simulink model "npc_controller"  (R2022a)
settings: Solver=FixedStepDiscrete  StartTime=0.0  StopTime=20  RelTol=1e-3  EnableMultiTasking=on
values from neighbouring files (symbols this model uses):
  Tsw = 1.5E-5    [param.sldd]
undefined symbols (not defined in the file or in its folder): CAN_O_INT, CANA_BASE, Down, GPTRIP1SEL, GPTRIP2SEL, GPTRIP3SEL, TZ1, TZ2, TZ3, Up
libraries: simulink x153, hdlsllib x90, c2802xlib x34, c2837xDlib x18, c280xlib x12, canmsglib x9, c2838xlib x8, idelinklib_common x3, c2806xlib x2, slpidlib x2, c28004xlib x2, c281xlib x2
(part 27 of 45)

== system npc_controller/CONTROL/STATE-MACHINE/CPU_CONTROL_750_A2_precharge_pfc_ok2_OL SS1/updateSequencePhA/pol_final1/pol_vxn ==
  vxn : Inport
  Action Port : ActionPort
  Out1 : Outport
  wires:
  vxn/1 -> Out1/1

== system npc_controller/CONTROL/STATE-MACHINE/CPU_CONTROL_750_A2_precharge_pfc_ok2_OL SS1/updateSequencePhA/pol_final1/prot ==
  note: Note:
      |
      | Function PWM # GPIO # LAUNCHPAD PIN #
      |
      | Synci EPWM1A GPIO0 J4.40
      | EPWM1B GPIO1 J4.39
      |
      | TZ GPIO62 XX
      |
      | a_s1 EPWM6B GPIO11 J8.75
      | a_s2 EPWM7B GPIO13 XX
      | a_s3 EPWM6A GPIO10 J8.76
      | a_s4 EPWM7A GPIO12 XX
      |
      | b_s1 EPWM8B GPIO15 J8.73
      | b_s2 EPWM9B GPIO17 XX
      | b_s3 EPWM8A GPIO14 J8.74
      | b_s4 EPWM9A GPIO16 J4.33
      |
      | c_s1 EPWM10B GPIO19 J1.3
      | c_s2 EPWM11B GPIO21 XX
      | c_s3 EPWM10A GPIO18 J1.4
      | c_s4 EPWM11A GPIO20 XX
  note: /*Force PWM to LOW*/
      | EPwm6Regs.AQCSFRC.bit.CSFA = (uint16_T)(0b01);
      | EPwm6Regs.AQCSFRC.bit.CSFB = (uint16_T)(0b01);
      | EPwm7Regs.AQCSFRC.bit.CSFA = (uint16_T)(0b01);
      | EPwm7Regs.AQCSFRC.bit.CSFB = (uint16_T)(0b01);
      | EPwm8Regs.AQCSFRC.bit.CSFA = (uint16_T)(0b01);
      | EPwm8Regs.AQCSFRC.bit.CSFB = (uint16_T)(0b01);
      | EPwm9Regs.AQCSFRC.bit.CSFA = (uint16_T)(0b01);
      | EPwm9Regs.AQCSFRC.bit.CSFB = (uint16_T)(0b01);
      | EPwm10Regs.AQCSFRC.bit.CSFA = (uint16_T)(0b01);
      | EPwm10Regs.AQCSFRC.bit.CSFB = (uint16_T)(0b01);
      | EPwm11Regs.AQCSFRC.bit.CSFA = (uint16_T)(0b01);
      | EPwm11Regs.AQCSFRC.bit.CSFB = (uint16_T)(0b01);
  note: Note:
      | AQCSFRC
      | 0b00 - disables forced PWM
      | 0b01 - forces PWM to LOW
      | 0b10 - forces PWM to  HIGH
  Action Port : ActionPort
  Constant : Constant  Value=0  OutDataTypeStr=uint8  SampleTime=-1
  System Outputs : Subsystem  mask(System Outputs){ShowInLibBrowser=0}
      mask prompts: ShowInLibBrowser "Simulink:masks:CustCodeMaskParam1_MP"
      settings: CopyFcn=cccopyfcn(gcb)  OpenFcn=ccopenfcn('System Outputs Function')
      mask Help: eval('feval(''rtwprivate'',''rtwhelpview'',''rtw_sys_outputs_block'')');
      mask Display: disp('System\nOutputs');
  Out1 : Outport
  wires:
  Constant/1 -> Out1/1

== system npc_controller/CONTROL/STATE-MACHINE/CPU_CONTROL_750_A2_precharge_pfc_ok2_OL SS1/updateSequencePhA/pol_ix1/neg ==
  Action Port : ActionPort
  Constant : Constant  Value=2  OutDataTypeStr=uint8  SampleTime=-1
  Out1 : Outport
  wires:
  Constant/1 -> Out1/1

== system npc_controller/CONTROL/STATE-MACHINE/CPU_CONTROL_750_A2_precharge_pfc_ok2_OL SS1/updateSequencePhA/pol_ix1/pos ==
  Action Port : ActionPort
  Constant : Constant  OutDataTypeStr=uint8  SampleTime=-1
  Out1 : Outport
  wires:
  Constant/1 -> Out1/1

== system npc_controller/CONTROL/STATE-MACHINE/CPU_CONTROL_750_A2_precharge_pfc_ok2_OL SS1/updateSequencePhA/pol_ix1/zero ==
  Action Port : ActionPort
  Constant : Constant  Value=0  OutDataTypeStr=uint8  SampleTime=-1
  Out1 : Outport
  wires:
  Constant/1 -> Out1/1

== system npc_controller/CONTROL/STATE-MACHINE/CPU_CONTROL_750_A2_precharge_pfc_ok2_OL SS1/updateSequencePhA/pol_vxn1/neg ==
  note: EPwm2Regs.AQCSFRC.bit.CSFA = (uint16_T)(0b01);
      | EPwm7Regs.AQCSFRC.bit.CSFB = (uint16_T)(0b00);
      | EPwm2Regs.AQCSFRC.bit.CSFB = (uint16_T)(0b10);
      | EPwm7Regs.AQCSFRC.bit.CSFA = (uint16_T)(0b01);
  note: Note:
      | AQCSFRC
      | 0b00 - disables forced PWM
      | 0b01 - forces PWM to LOW
      | 0b10 - forces PWM to  HIGH
  note: Note:
      |
      | Function PWM # GPIO # LAUNCHPAD PIN #
      |
      | Synci EPWM1A GPIO0 J4.40
      | EPWM1B GPIO1 J4.39
      |
      | ORPS EPMW2A GPIO2 J4.38
      | EPWM2B GPIO3 J4.37
      |
      | RELAY EPWM3A GPIO4 J4.36
      |
      | TZ GPIO62 XX
      |
      | a_s1 EPWM6A GPIO10 J8.76
      | a_s2 EPWM7B GPIO13 XX
      | a_s3 EPWM6B GPIO11 J8.75
      | a_s4 EPWM7A GPIO12 XX
      |
      | b_s1 EPWM8B GPIO15 J8.73
      | b_s2 EPWM9B GPIO17 XX
      | b_s3 EPWM8A GPIO14 J8.74
      | b_s4 EPWM9A GPIO16 J4.33
      |
      | c_s1 EPWM10B GPIO19 J1.3
      | c_s2 EPWM11B GPIO21 XX
      | c_s3 EPWM10A GPIO18 J1.4
      | c_s4 EPWM11A GPIO20 XX
  Action Port : ActionPort
  Constant : Constant  Value=2  OutDataTypeStr=uint8  SampleTime=-1
  System Outputs1 : Subsystem  mask(System Outputs){ShowInLibBrowser=0}
      mask prompts: ShowInLibBrowser "Simulink:masks:CustCodeMaskParam1_MP"
      settings: CopyFcn=cccopyfcn(gcb)  OpenFcn=ccopenfcn('System Outputs Function')
      mask Help: eval('feval(''rtwprivate'',''rtwhelpview'',''rtw_sys_outputs_block'')');
      mask Display: disp('System\nOutputs');
  Out1 : Outport
  wires:
  Constant/1 -> Out1/1

== system npc_controller/CONTROL/STATE-MACHINE/CPU_CONTROL_750_A2_precharge_pfc_ok2_OL SS1/updateSequencePhA/pol_vxn1/pos ==
  note: Note:
      | AQCSFRC
      | 0b00 - disables forced PWM
      | 0b01 - forces PWM to LOW
      | 0b10 - forces PWM to  HIGH
  note: EPwm2Regs.AQCSFRC.bit.CSFA = (uint16_T)(0b01);
      | EPwm7Regs.AQCSFRC.bit.CSFB = (uint16_T)(0b10);
      | EPwm2Regs.AQCSFRC.bit.CSFB = (uint16_T)(0b00);
      | EPwm7Regs.AQCSFRC.bit.CSFA = (uint16_T)(0b01);
  note: Note:
      |
      | Function PWM # GPIO # LAUNCHPAD PIN #
      |
      | Synci EPWM1A GPIO0 J4.40
      | EPWM1B GPIO1 J4.39
      |
      | ORPS EPMW2A GPIO2 J4.38
      | EPWM2B GPIO3 J4.37
      |
      | RELAY EPWM3A GPIO4 J4.36
      |
      | TZ GPIO62 XX
      |
      | a_s1 EPWM6A GPIO10 J8.76
      | a_s2 EPWM7B GPIO13 XX
      | a_s3 EPWM6B GPIO11 J8.75
      | a_s4 EPWM7A GPIO12 XX
      |
      | b_s1 EPWM8B GPIO15 J8.73
      | b_s2 EPWM9B GPIO17 XX
      | b_s3 EPWM8A GPIO14 J8.74
      | b_s4 EPWM9A GPIO16 J4.33
      |
      | c_s1 EPWM10B GPIO19 J1.3
      | c_s2 EPWM11B GPIO21 XX
      | c_s3 EPWM10A GPIO18 J1.4
      | c_s4 EPWM11A GPIO20 XX
  Action Port : ActionPort
  Constant : Constant  OutDataTypeStr=uint8  SampleTime=-1
  System Outputs1 : Subsystem  mask(System Outputs){ShowInLibBrowser=0}
      mask prompts: ShowInLibBrowser "Simulink:masks:CustCodeMaskParam1_MP"
      settings: CopyFcn=cccopyfcn(gcb)  OpenFcn=ccopenfcn('System Outputs Function')
      mask Help: eval('feval(''rtwprivate'',''rtwhelpview'',''rtw_sys_outputs_block'')');
      mask Display: disp('System\nOutputs');
  Out1 : Outport
  wires:
  Constant/1 -> Out1/1

== system npc_controller/CONTROL/STATE-MACHINE/CPU_CONTROL_750_A2_precharge_pfc_ok2_OL SS1/updateSequencePhA/pol_vxn1/zero ==
  note: /*Force PWM to LOW*/
      | EPwm2Regs.AQCSFRC.bit.CSFA = (uint16_T)(0b01);
      | EPwm7Regs.AQCSFRC.bit.CSFB = (uint16_T)(0b01);
      | EPwm2Regs.AQCSFRC.bit.CSFB = (uint16_T)(0b01);
      | EPwm7Regs.AQCSFRC.bit.CSFA = (uint16_T)(0b01);
  note: Note:
      | AQCSFRC
      | 0b00 - disables forced PWM
      | 0b01 - forces PWM to LOW
      | 0b10 - forces PWM to  HIGH
  note: Note:
      |
      | Function PWM # GPIO # LAUNCHPAD PIN #
      |
      | Synci EPWM1A GPIO0 J4.40
      | EPWM1B GPIO1 J4.39
      |
      | ORPS EPMW2A GPIO2 J4.38
      | EPWM2B GPIO3 J4.37
      |
      | RELAY EPWM3A GPIO4 J4.36
      |
      | TZ GPIO62 XX
      |
      | a_s1 EPWM6A GPIO10 J8.76
      | a_s2 EPWM7B GPIO13 XX
      | a_s3 EPWM6B GPIO11 J8.75
      | a_s4 EPWM7A GPIO12 XX
      |
      | b_s1 EPWM8B GPIO15 J8.73
      | b_s2 EPWM9B GPIO17 XX
      | b_s3 EPWM8A GPIO14 J8.74
      | b_s4 EPWM9A GPIO16 J4.33
      |
      | c_s1 EPWM10B GPIO19 J1.3
      | c_s2 EPWM11B GPIO21 XX
      | c_s3 EPWM10A GPIO18 J1.4
      | c_s4 EPWM11A GPIO20 XX
  Action Port : ActionPort
  Constant : Constant  Value=0  OutDataTypeStr=uint8  SampleTime=-1
  System Outputs1 : Subsystem  mask(System Outputs){ShowInLibBrowser=0}
      mask prompts: ShowInLibBrowser "Simulink:masks:CustCodeMaskParam1_MP"
      settings: CopyFcn=cccopyfcn(gcb)  OpenFcn=ccopenfcn('System Outputs Function')
      mask Help: eval('feval(''rtwprivate'',''rtwhelpview'',''rtw_sys_outputs_block'')');
      mask Display: disp('System\nOutputs');
  Out1 : Outport
  wires:
  Constant/1 -> Out1/1

== system npc_controller/CONTROL/STATE-MACHINE/CPU_CONTROL_750_A2_precharge_pfc_ok2_OL SS1/updateSequencePhB/pol_final1/pol_vxn ==
  vxn : Inport
  Action Port : ActionPort
  Out1 : Outport
  wires:
  vxn/1 -> Out1/1

== system npc_controller/CONTROL/STATE-MACHINE/CPU_CONTROL_750_A2_precharge_pfc_ok2_OL SS1/updateSequencePhB/pol_final1/prot ==
  note: Note:
      |
      | Function PWM # GPIO # LAUNCHPAD PIN #
      |
      | Synci EPWM1A GPIO0 J4.40
      | EPWM1B GPIO1 J4.39
      |
      | TZ GPIO62 XX
      |
      | a_s1 EPWM6B GPIO11 J8.75
      | a_s2 EPWM7B GPIO13 XX
      | a_s3 EPWM6A GPIO10 J8.76
      | a_s4 EPWM7A GPIO12 XX
      |
      | b_s1 EPWM8B GPIO15 J8.73
      | b_s2 EPWM9B GPIO17 XX
      | b_s3 EPWM8A GPIO14 J8.74
      | b_s4 EPWM9A GPIO16 J4.33
      |
      | c_s1 EPWM10B GPIO19 J1.3
      | c_s2 EPWM11B GPIO21 XX
      | c_s3 EPWM10A GPIO18 J1.4
      | c_s4 EPWM11A GPIO20 XX
  note: /*Force PWM to LOW*/
      | EPwm6Regs.AQCSFRC.bit.CSFA = (uint16_T)(0b01);
      | EPwm6Regs.AQCSFRC.bit.CSFB = (uint16_T)(0b01);
      | EPwm7Regs.AQCSFRC.bit.CSFA = (uint16_T)(0b01);
      | EPwm7Regs.AQCSFRC.bit.CSFB = (uint16_T)(0b01);
      | EPwm8Regs.AQCSFRC.bit.CSFA = (uint16_T)(0b01);
      | EPwm8Regs.AQCSFRC.bit.CSFB = (uint16_T)(0b01);
      | EPwm9Regs.AQCSFRC.bit.CSFA = (uint16_T)(0b01);
      | EPwm9Regs.AQCSFRC.bit.CSFB = (uint16_T)(0b01);
      | EPwm10Regs.AQCSFRC.bit.CSFA = (uint16_T)(0b01);
      | EPwm10Regs.AQCSFRC.bit.CSFB = (uint16_T)(0b01);
      | EPwm11Regs.AQCSFRC.bit.CSFA = (uint16_T)(0b01);
      | EPwm11Regs.AQCSFRC.bit.CSFB = (uint16_T)(0b01);
  note: Note:
      | AQCSFRC
      | 0b00 - disables forced PWM
      | 0b01 - forces PWM to LOW
      | 0b10 - forces PWM to  HIGH
  Action Port : ActionPort
  Constant : Constant  Value=0  OutDataTypeStr=uint8  SampleTime=-1
  System Outputs : Subsystem  mask(System Outputs){ShowInLibBrowser=0}
      mask prompts: ShowInLibBrowser "Simulink:masks:CustCodeMaskParam1_MP"
      settings: CopyFcn=cccopyfcn(gcb)  OpenFcn=ccopenfcn('System Outputs Function')
      mask Help: eval('feval(''rtwprivate'',''rtwhelpview'',''rtw_sys_outputs_block'')');
      mask Display: disp('System\nOutputs');
  Out1 : Outport
  wires:
  Constant/1 -> Out1/1

== system npc_controller/CONTROL/STATE-MACHINE/CPU_CONTROL_750_A2_precharge_pfc_ok2_OL SS1/updateSequencePhB/pol_ix1/neg ==
  Action Port : ActionPort
  Constant : Constant  Value=2  OutDataTypeStr=uint8  SampleTime=-1
  Out1 : Outport
  wires:
  Constant/1 -> Out1/1

== system npc_controller/CONTROL/STATE-MACHINE/CPU_CONTROL_750_A2_precharge_pfc_ok2_OL SS1/updateSequencePhB/pol_ix1/pos ==
  Action Port : ActionPort
  Constant : Constant  OutDataTypeStr=uint8  SampleTime=-1
  Out1 : Outport
  wires:
  Constant/1 -> Out1/1

== system npc_controller/CONTROL/STATE-MACHINE/CPU_CONTROL_750_A2_precharge_pfc_ok2_OL SS1/updateSequencePhB/pol_ix1/zero ==
  Action Port : ActionPort
  Constant : Constant  Value=0  OutDataTypeStr=uint8  SampleTime=-1
  Out1 : Outport
  wires:
  Constant/1 -> Out1/1

== system npc_controller/CONTROL/STATE-MACHINE/CPU_CONTROL_750_A2_precharge_pfc_ok2_OL SS1/updateSequencePhB/pol_vxn1/neg ==
  note: Note:
      |
      | Function PWM # GPIO # LAUNCHPAD PIN #
      |
      | Synci EPWM1A GPIO0 J4.40
      | EPWM1B GPIO1 J4.39
      |
      | TZ GPIO62 XX
      |
      | a_s1 EPWM6B GPIO11 J8.75
      | a_s2 EPWM7B GPIO13 XX
      | a_s3 EPWM6A GPIO10 J8.76
      | a_s4 EPWM7A GPIO12 XX
      |
      | b_s1 EPWM8B GPIO15 J8.73
      | b_s2 EPWM9B GPIO17 XX
      | b_s3 EPWM8A GPIO14 J8.74
      | b_s4 EPWM9A GPIO16 J4.33
      |
      | c_s1 EPWM10B GPIO19 J1.3
      | c_s2 EPWM11B GPIO21 XX
      | c_s3 EPWM10A GPIO18 J1.4
      | c_s4 EPWM11A GPIO20 XX
  note: Note:
      | AQCSFRC
      | 0b00 - disables forced PWM
      | 0b01 - forces PWM to LOW
      | 0b10 - forces PWM to  HIGH
  note: EPwm8Regs.AQCSFRC.bit.CSFB = (uint16_T)(0b01);
      | EPwm9Regs.AQCSFRC.bit.CSFB = (uint16_T)(0b00);
      | EPwm8Regs.AQCSFRC.bit.CSFA = (uint16_T)(0b10);
      | EPwm9Regs.AQCSFRC.bit.CSFA = (uint16_T)(0b01);
  Action Port : ActionPort
  Constant : Constant  Value=2  OutDataTypeStr=uint8  SampleTime=-1
  System Outputs1 : Subsystem  mask(System Outputs){ShowInLibBrowser=0}
      mask prompts: ShowInLibBrowser "Simulink:masks:CustCodeMaskParam1_MP"
      settings: CopyFcn=cccopyfcn(gcb)  OpenFcn=ccopenfcn('System Outputs Function')
      mask Help: eval('feval(''rtwprivate'',''rtwhelpview'',''rtw_sys_outputs_block'')');
      mask Display: disp('System\nOutputs');
  Out1 : Outport
  wires:
  Constant/1 -> Out1/1

== system npc_controller/CONTROL/STATE-MACHINE/CPU_CONTROL_750_A2_precharge_pfc_ok2_OL SS1/updateSequencePhB/pol_vxn1/pos ==
  note: Note:
      | AQCSFRC
      | 0b00 - disables forced PWM
      | 0b01 - forces PWM to LOW
      | 0b10 - forces PWM to  HIGH
  note: Note:
      |
      | Function PWM # GPIO # LAUNCHPAD PIN #
      |
      | Synci EPWM1A GPIO0 J4.40
      | EPWM1B GPIO1 J4.39
      |
      | TZ GPIO62 XX
      |
      | a_s1 EPWM6B GPIO11 J8.75
      | a_s2 EPWM7B GPIO13 XX
      | a_s3 EPWM6A GPIO10 J8.76
      | a_s4 EPWM7A GPIO12 XX
      |
      | b_s1 EPWM8B GPIO15 J8.73
      | b_s2 EPWM9B GPIO17 XX
      | b_s3 EPWM8A GPIO14 J8.74
      | b_s4 EPWM9A GPIO16 J4.33
      |
      | c_s1 EPWM10B GPIO19 J1.3
      | c_s2 EPWM11B GPIO21 XX
      | c_s3 EPWM10A GPIO18 J1.4
      | c_s4 EPWM11A GPIO20 XX
  note: EPwm8Regs.AQCSFRC.bit.CSFB = (uint16_T)(0b01);
      | EPwm9Regs.AQCSFRC.bit.CSFB = (uint16_T)(0b10);
      | EPwm8Regs.AQCSFRC.bit.CSFA = (uint16_T)(0b00);
      | EPwm9Regs.AQCSFRC.bit.CSFA = (uint16_T)(0b01);
  Action Port : ActionPort
  Constant : Constant  OutDataTypeStr=uint8  SampleTime=-1
  System Outputs1 : Subsystem  mask(System Outputs){ShowInLibBrowser=0}
      mask prompts: ShowInLibBrowser "Simulink:masks:CustCodeMaskParam1_MP"
      settings: CopyFcn=cccopyfcn(gcb)  OpenFcn=ccopenfcn('System Outputs Function')
      mask Help: eval('feval(''rtwprivate'',''rtwhelpview'',''rtw_sys_outputs_block'')');
      mask Display: disp('System\nOutputs');
  Out1 : Outport
  wires:
  Constant/1 -> Out1/1

== system npc_controller/CONTROL/STATE-MACHINE/CPU_CONTROL_750_A2_precharge_pfc_ok2_OL SS1/updateSequencePhB/pol_vxn1/zero ==
  note: Note:
      |
      | Function PWM # GPIO # LAUNCHPAD PIN #
      |
      | Synci EPWM1A GPIO0 J4.40
      | EPWM1B GPIO1 J4.39
      |
      | TZ GPIO62 XX
      |
      | a_s1 EPWM6B GPIO11 J8.75
      | a_s2 EPWM7B GPIO13 XX
      | a_s3 EPWM6A GPIO10 J8.76
      | a_s4 EPWM7A GPIO12 XX
      |
      | b_s1 EPWM8B GPIO15 J8.73
      | b_s2 EPWM9B GPIO17 XX
      | b_s3 EPWM8A GPIO14 J8.74
      | b_s4 EPWM9A GPIO16 J4.33
      |
      | c_s1 EPWM10B GPIO19 J1.3
      | c_s2 EPWM11B GPIO21 XX
      | c_s3 EPWM10A GPIO18 J1.4
      | c_s4 EPWM11A GPIO20 XX
  note: /*Force PWM to LOW*/
      | EPwm8Regs.AQCSFRC.bit.CSFB = (uint16_T)(0b01);
      | EPwm9Regs.AQCSFRC.bit.CSFB = (uint16_T)(0b01);
      | EPwm8Regs.AQCSFRC.bit.CSFA = (uint16_T)(0b01);
      | EPwm9Regs.AQCSFRC.bit.CSFA = (uint16_T)(0b01);
  note: Note:
      | AQCSFRC
      | 0b00 - disables forced PWM
      | 0b01 - forces PWM to LOW
      | 0b10 - forces PWM to  HIGH
  Action Port : ActionPort
  Constant : Constant  Value=0  OutDataTypeStr=uint8  SampleTime=-1
  System Outputs1 : Subsystem  mask(System Outputs){ShowInLibBrowser=0}
      mask prompts: ShowInLibBrowser "Simulink:masks:CustCodeMaskParam1_MP"
      settings: CopyFcn=cccopyfcn(gcb)  OpenFcn=ccopenfcn('System Outputs Function')
      mask Help: eval('feval(''rtwprivate'',''rtwhelpview'',''rtw_sys_outputs_block'')');
      mask Display: disp('System\nOutputs');
  Out1 : Outport
  wires:
  Constant/1 -> Out1/1

== system npc_controller/CONTROL/STATE-MACHINE/CPU_CONTROL_750_A2_precharge_pfc_ok2_OL SS1/updateSequencePhC/pol_final1/pol_vxn ==
  vxn : Inport
  Action Port : ActionPort
  Out1 : Outport
  wires:
  vxn/1 -> Out1/1

== system npc_controller/CONTROL/STATE-MACHINE/CPU_CONTROL_750_A2_precharge_pfc_ok2_OL SS1/updateSequencePhC/pol_final1/prot ==
  note: Note:
      |
      | Function PWM # GPIO # LAUNCHPAD PIN #
      |
      | Synci EPWM1A GPIO0 J4.40
      | EPWM1B GPIO1 J4.39
      |
      | TZ GPIO62 XX
      |
      | a_s1 EPWM6B GPIO11 J8.75
      | a_s2 EPWM7B GPIO13 XX
      | a_s3 EPWM6A GPIO10 J8.76
      | a_s4 EPWM7A GPIO12 XX
      |
      | b_s1 EPWM8B GPIO15 J8.73
      | b_s2 EPWM9B GPIO17 XX
      | b_s3 EPWM8A GPIO14 J8.74
      | b_s4 EPWM9A GPIO16 J4.33
      |
      | c_s1 EPWM10B GPIO19 J1.3
      | c_s2 EPWM11B GPIO21 XX
      | c_s3 EPWM10A GPIO18 J1.4
      | c_s4 EPWM11A GPIO20 XX
  note: /*Force PWM to LOW*/
      | EPwm6Regs.AQCSFRC.bit.CSFA = (uint16_T)(0b01);
      | EPwm6Regs.AQCSFRC.bit.CSFB = (uint16_T)(0b01);
      | EPwm7Regs.AQCSFRC.bit.CSFA = (uint16_T)(0b01);
      | EPwm7Regs.AQCSFRC.bit.CSFB = (uint16_T)(0b01);
      | EPwm8Regs.AQCSFRC.bit.CSFA = (uint16_T)(0b01);
      | EPwm8Regs.AQCSFRC.bit.CSFB = (uint16_T)(0b01);
      | EPwm9Regs.AQCSFRC.bit.CSFA = (uint16_T)(0b01);
      | EPwm9Regs.AQCSFRC.bit.CSFB = (uint16_T)(0b01);
      | EPwm10Regs.AQCSFRC.bit.CSFA = (uint16_T)(0b01);
      | EPwm10Regs.AQCSFRC.bit.CSFB = (uint16_T)(0b01);
      | EPwm11Regs.AQCSFRC.bit.CSFA = (uint16_T)(0b01);
      | EPwm11Regs.AQCSFRC.bit.CSFB = (uint16_T)(0b01);
  note: Note:
      | AQCSFRC
      | 0b00 - disables forced PWM
      | 0b01 - forces PWM to LOW
      | 0b10 - forces PWM to  HIGH
  Action Port : ActionPort
  Constant : Constant  Value=0  OutDataTypeStr=uint8  SampleTime=-1
  System Outputs : Subsystem  mask(System Outputs){ShowInLibBrowser=0}
      mask prompts: ShowInLibBrowser "Simulink:masks:CustCodeMaskParam1_MP"
      settings: CopyFcn=cccopyfcn(gcb)  OpenFcn=ccopenfcn('System Outputs Function')
      mask Help: eval('feval(''rtwprivate'',''rtwhelpview'',''rtw_sys_outputs_block'')');
      mask Display: disp('System\nOutputs');
  Out1 : Outport
  wires:
  Constant/1 -> Out1/1

== system npc_controller/CONTROL/STATE-MACHINE/CPU_CONTROL_750_A2_precharge_pfc_ok2_OL SS1/updateSequencePhC/pol_ix1/neg ==
  Action Port : ActionPort
  Constant : Constant  Value=2  OutDataTypeStr=uint8  SampleTime=-1
  Out1 : Outport
  wires:
  Constant/1 -> Out1/1

== system npc_controller/CONTROL/STATE-MACHINE/CPU_CONTROL_750_A2_precharge_pfc_ok2_OL SS1/updateSequencePhC/pol_ix1/pos ==
  Action Port : ActionPort
  Constant : Constant  OutDataTypeStr=uint8  SampleTime=-1
  Out1 : Outport
  wires:
  Constant/1 -> Out1/1

== system npc_controller/CONTROL/STATE-MACHINE/CPU_CONTROL_750_A2_precharge_pfc_ok2_OL SS1/updateSequencePhC/pol_ix1/zero ==
  Action Port : ActionPort
  Constant : Constant  Value=0  OutDataTypeStr=uint8  SampleTime=-1
  Out1 : Outport
  wires:
  Constant/1 -> Out1/1

== system npc_controller/CONTROL/STATE-MACHINE/CPU_CONTROL_750_A2_precharge_pfc_ok2_OL SS1/updateSequencePhC/pol_vxn1/neg ==
  note: Note:
      | AQCSFRC
      | 0b00 - disables forced PWM
      | 0b01 - forces PWM to LOW
      | 0b10 - forces PWM to  HIGH
  note: EPwm10Regs.AQCSFRC.bit.CSFB = (uint16_T)(0b01);
      | EPwm11Regs.AQCSFRC.bit.CSFB = (uint16_T)(0b00);
      | EPwm10Regs.AQCSFRC.bit.CSFA = (uint16_T)(0b10);
      | EPwm11Regs.AQCSFRC.bit.CSFA = (uint16_T)(0b01);
  note: Note:
      |
      | Function PWM # GPIO # LAUNCHPAD PIN #
      |
      | Synci EPWM1A GPIO0 J4.40
      | EPWM1B GPIO1 J4.39
      |
      | TZ GPIO62 XX
      |
      | a_s1 EPWM6B GPIO11 J8.75
      | a_s2 EPWM7B GPIO13 XX
      | a_s3 EPWM6A GPIO10 J8.76
      | a_s4 EPWM7A GPIO12 XX
      |
      | b_s1 EPWM8B GPIO15 J8.73
      | b_s2 EPWM9B GPIO17 XX
      | b_s3 EPWM8A GPIO14 J8.74
      | b_s4 EPWM9A GPIO16 J4.33
      |
      | c_s1 EPWM10B GPIO19 J1.3
      | c_s2 EPWM11B GPIO21 XX
      | c_s3 EPWM10A GPIO18 J1.4
      | c_s4 EPWM11A GPIO20 XX
  Action Port : ActionPort
  Constant : Constant  Value=2  OutDataTypeStr=uint8  SampleTime=-1
  System Outputs1 : Subsystem  mask(System Outputs){ShowInLibBrowser=0}
      mask prompts: ShowInLibBrowser "Simulink:masks:CustCodeMaskParam1_MP"
      settings: CopyFcn=cccopyfcn(gcb)  OpenFcn=ccopenfcn('System Outputs Function')
      mask Help: eval('feval(''rtwprivate'',''rtwhelpview'',''rtw_sys_outputs_block'')');
      mask Display: disp('System\nOutputs');
  Out1 : Outport
  wires:
  Constant/1 -> Out1/1

== system npc_controller/CONTROL/STATE-MACHINE/CPU_CONTROL_750_A2_precharge_pfc_ok2_OL SS1/updateSequencePhC/pol_vxn1/pos ==
  note: EPwm10Regs.AQCSFRC.bit.CSFB = (uint16_T)(0b01);
      | EPwm11Regs.AQCSFRC.bit.CSFB = (uint16_T)(0b10);
      | EPwm10Regs.AQCSFRC.bit.CSFA = (uint16_T)(0b00);
      | EPwm11Regs.AQCSFRC.bit.CSFA = (uint16_T)(0b01);
  note: Note:
      |
      | Function PWM # GPIO # LAUNCHPAD PIN #
      |
      | Synci EPWM1A GPIO0 J4.40
      | EPWM1B GPIO1 J4.39
      |
      | TZ GPIO62 XX
      |
      | a_s1 EPWM6B GPIO11 J8.75
      | a_s2 EPWM7B GPIO13 XX
      | a_s3 EPWM6A GPIO10 J8.76
      | a_s4 EPWM7A GPIO12 XX
      |
      | b_s1 EPWM8B GPIO15 J8.73
      | b_s2 EPWM9B GPIO17 XX
      | b_s3 EPWM8A GPIO14 J8.74
      | b_s4 EPWM9A GPIO16 J4.33
      |
      | c_s1 EPWM10B GPIO19 J1.3
      | c_s2 EPWM11B GPIO21 XX
      | c_s3 EPWM10A GPIO18 J1.4
      | c_s4 EPWM11A GPIO20 XX
  note: Note:
      | AQCSFRC
      | 0b00 - disables forced PWM
      | 0b01 - forces PWM to LOW
      | 0b10 - forces PWM to  HIGH
  Action Port : ActionPort
  Constant : Constant  OutDataTypeStr=uint8  SampleTime=-1
  System Outputs1 : Subsystem  mask(System Outputs){ShowInLibBrowser=0}
      mask prompts: ShowInLibBrowser "Simulink:masks:CustCodeMaskParam1_MP"
      settings: CopyFcn=cccopyfcn(gcb)  OpenFcn=ccopenfcn('System Outputs Function')
      mask Help: eval('feval(''rtwprivate'',''rtwhelpview'',''rtw_sys_outputs_block'')');
      mask Display: disp('System\nOutputs');
  Out1 : Outport
  wires:
  Constant/1 -> Out1/1

== system npc_controller/CONTROL/STATE-MACHINE/CPU_CONTROL_750_A2_precharge_pfc_ok2_OL SS1/updateSequencePhC/pol_vxn1/zero ==
  note: Note:
      | AQCSFRC
      | 0b00 - disables forced PWM
      | 0b01 - forces PWM to LOW
      | 0b10 - forces PWM to  HIGH
  note: /*Force PWM to LOW*/
      | EPwm10Regs.AQCSFRC.bit.CSFB = (uint16_T)(0b01);
      | EPwm11Regs.AQCSFRC.bit.CSFB = (uint16_T)(0b01);
      | EPwm10Regs.AQCSFRC.bit.CSFA = (uint16_T)(0b01);
      | EPwm11Regs.AQCSFRC.bit.CSFA = (uint16_T)(0b01);
  note: Note:
      |
      | Function PWM # GPIO # LAUNCHPAD PIN #
      |
      | Synci EPWM1A GPIO0 J4.40
      | EPWM1B GPIO1 J4.39
      |
      | TZ GPIO62 XX
      |
      | a_s1 EPWM6B GPIO11 J8.75
      | a_s2 EPWM7B GPIO13 XX
      | a_s3 EPWM6A GPIO10 J8.76
      | a_s4 EPWM7A GPIO12 XX
      |
      | b_s1 EPWM8B GPIO15 J8.73
      | b_s2 EPWM9B GPIO17 XX
      | b_s3 EPWM8A GPIO14 J8.74
      | b_s4 EPWM9A GPIO16 J4.33
      |
      | c_s1 EPWM10B GPIO19 J1.3
      | c_s2 EPWM11B GPIO21 XX
      | c_s3 EPWM10A GPIO18 J1.4
      | c_s4 EPWM11A GPIO20 XX
  Action Port : ActionPort
  Constant : Constant  Value=0  OutDataTypeStr=uint8  SampleTime=-1
  System Outputs1 : Subsystem  mask(System Outputs){ShowInLibBrowser=0}
      mask prompts: ShowInLibBrowser "Simulink:masks:CustCodeMaskParam1_MP"
      settings: CopyFcn=cccopyfcn(gcb)  OpenFcn=ccopenfcn('System Outputs Function')
      mask Help: eval('feval(''rtwprivate'',''rtwhelpview'',''rtw_sys_outputs_block'')');
      mask Display: disp('System\nOutputs');
  Out1 : Outport
  wires:
  Constant/1 -> Out1/1

== system npc_controller/CONTROL/STATE-MACHINE/CPU_CONTROL_750_A2_precharge_pfc_ok2_OL SS2/configGrid/FORCE_TZ/1P ==
  note: 1 - Leg A
      | 2 - Leg B
      | 3 - Leg C
      | 4 - All legs
  sinlgeph_config : Inport
  Action Port : ActionPort
  ALL_LEGS : Subsystem  Commented=on  TreatAsAtomicUnit=on
  If : If  IfExpression=u1 == 1  ElseIfExpressions=u1 == 2, u1 == 3, u1 == 4
  LEG_A : Subsystem  TreatAsAtomicUnit=on
  LEG_B : Subsystem  TreatAsAtomicUnit=on
  LEG_C : Subsystem  TreatAsAtomicUnit=on
  wires:
  If/4 -> ALL_LEGS/Action
  If/3 -> LEG_C/Action
  If/2 -> LEG_B/Action
  sinlgeph_config/1 -> If/1
  If/1 -> LEG_A/Action

== system npc_controller/CONTROL/STATE-MACHINE/CPU_CONTROL_750_A2_precharge_pfc_ok2_OL SS2/configGrid/FORCE_TZ/3P3W ==
  note: Note:
      | TZCCTL
      | 0b00 - High impedance
      | 0b01 - Force to HIGH
      | 0b10 - Force to LOW
      | 0b11 - Do nothing
      |
      | AQCSFRC
      | 0b00 - disables forced PWM
      | 0b01 - forces PWM to LOW
      | 0b10 - forces PWM to  HIGH
      |
      | TZFRC.bit.OST
      | 0b0 - Do nothing
      | 0b1 - Force TZ
  note: EALLOW;
      |
      | /*Force TZ*/
      | EPwm6Regs. TZFRC.bit.OST = 0b0; //do nothing
      | EPwm7Regs. TZFRC.bit.OST = 0b0;
      | EPwm8Regs. TZFRC.bit.OST = 0b0;
      | EPwm9Regs. TZFRC.bit.OST = 0b0;
      | EPwm10Regs. TZFRC.bit.OST = 0b0;
      | EPwm11Regs. TZFRC.bit.OST = 0b0;
      |
      | EDIS;
  Action Port : ActionPort
  System Outputs2 : Subsystem  mask(System Outputs){ShowInLibBrowser=0}
      mask prompts: ShowInLibBrowser "Simulink:masks:CustCodeMaskParam1_MP"
      settings: CopyFcn=cccopyfcn(gcb)  OpenFcn=ccopenfcn('System Outputs Function')
      mask Help: eval('feval(''rtwprivate'',''rtwhelpview'',''rtw_sys_outputs_block'')');
      mask Display: disp('System\nOutputs');

== system npc_controller/CONTROL/STATE-MACHINE/CPU_CONTROL_750_A2_precharge_pfc_ok2_OL SS2/configGrid/RESET_TZ/System Outputs2 ==

== system npc_controller/CONTROL/STATE-MACHINE/CPU_CONTROL_750_A2_precharge_pfc_ok2_OL SS2/updateCalib/cnt/IIR Filter2 ==
  note: prev 0.98
  x[n] : Inport
  1 - Lambda : Gain  Gain=1 - 0.95  ParamDataTypeStr=single  OutDataTypeStr=single
  Delay : Delay  DelayLength=1
  Lambda : Gain  Gain=0.95  ParamDataTypeStr=single  OutDataTypeStr=single
  Sum : Sum  Inputs=|++  AccumDataTypeStr=single  OutDataTypeStr=single
  y[n] : Outport
  wires:
  x[n]/1 -> 1 - Lambda/1
  1 - Lambda/1 -> Sum/1
  Sum/1 -> Delay/1, y[n]/1
  Lambda/1 -> Sum/2
  Delay/1 -> Lambda/1

== system npc_controller/CONTROL/STATE-MACHINE/CPU_CONTROL_750_A2_precharge_pfc_ok2_OL SS2/updateCalib/cnt/Subsystem1 ==
  sample : Inport
  Add4 : Sum  AccumDataTypeStr=single  OutDataTypeStr=single
  Cast To Single : DataTypeConversion  OutDataTypeStr=single  SaturateOnIntegerOverflow=off  RndMeth=Floor
  Constant4 : Constant  OutDataTypeStr=single
  Data Store Read4 : DataStoreRead  DataStoreName=cnt_calib  IndexOptions=Index vector (dialog)  Indices=1  OutputSizes=1
  Delay2 : Delay  DelayLength=1
  Divide3 : Product  Inputs=*/  OutDataTypeStr=single
  Divide4 : Product  Inputs=**/  OutDataTypeStr=single
  Subtract1 : Sum  Inputs=+-  AccumDataTypeStr=single  OutDataTypeStr=single
  average : Outport
  wires:
  Constant4/1 -> Subtract1/2
  Divide4/1 -> Add4/1
  Cast To Single/1 -> Subtract1/1, Divide4/3, Divide3/2
  Divide3/1 -> Add4/2
  Subtract1/1 -> Divide4/2
  Delay2/1 -> Divide4/1
  sample/1 -> Divide3/1
  Add4/1 -> average/1, Delay2/1
  Data Store Read4/1 -> Cast To Single/1

== system npc_controller/CONTROL/STATE-MACHINE/CPU_CONTROL_750_A2_precharge_pfc_ok2_OL SS2/updateCalib/cnt/Subsystem2 ==
  sample : Inport
  Add4 : Sum  AccumDataTypeStr=single  OutDataTypeStr=single
  Cast To Single : DataTypeConversion  OutDataTypeStr=single  SaturateOnIntegerOverflow=off  RndMeth=Floor
  Constant4 : Constant  OutDataTypeStr=single
  Data Store Read4 : DataStoreRead  DataStoreName=cnt_calib  IndexOptions=Index vector (dialog)  Indices=1  OutputSizes=1
  Delay2 : Delay  DelayLength=1
  Divide3 : Product  Inputs=*/  OutDataTypeStr=single
  Divide4 : Product  Inputs=**/  OutDataTypeStr=single
  Subtract1 : Sum  Inputs=+-  AccumDataTypeStr=single  OutDataTypeStr=single
  average : Outport
  wires:
  Data Store Read4/1 -> Cast To Single/1
  Add4/1 -> Delay2/1, average/1
  sample/1 -> Divide3/1
  Delay2/1 -> Divide4/1
  Subtract1/1 -> Divide4/2
  Divide3/1 -> Add4/2
  Cast To Single/1 -> Divide3/2, Divide4/3, Subtract1/1
  Divide4/1 -> Add4/1
  Constant4/1 -> Subtract1/2

== system npc_controller/CONTROL/STATE-MACHINE/CPU_CONTROL_750_A2_precharge_pfc_ok2_OL SS2/updateCalib/cnt/Subsystem3 ==
  sample : Inport
  Add4 : Sum  AccumDataTypeStr=single  OutDataTypeStr=single
  Cast To Single : DataTypeConversion  OutDataTypeStr=single  SaturateOnIntegerOverflow=off  RndMeth=Floor
  Constant4 : Constant  OutDataTypeStr=single
  Data Store Read4 : DataStoreRead  DataStoreName=cnt_calib  IndexOptions=Index vector (dialog)  Indices=1  OutputSizes=1
  Delay2 : Delay  DelayLength=1
  Divide3 : Product  Inputs=*/  OutDataTypeStr=single
  Divide4 : Product  Inputs=**/  OutDataTypeStr=single
  Subtract1 : Sum  Inputs=+-  AccumDataTypeStr=single  OutDataTypeStr=single
  average : Outport
  wires:
  Data Store Read4/1 -> Cast To Single/1
  Add4/1 -> Delay2/1, average/1
  sample/1 -> Divide3/1
  Delay2/1 -> Divide4/1
  Subtract1/1 -> Divide4/2
  Divide3/1 -> Add4/2
  Cast To Single/1 -> Divide3/2, Divide4/3, Subtract1/1
  Divide4/1 -> Add4/1
  Constant4/1 -> Subtract1/2

== system npc_controller/CONTROL/STATE-MACHINE/CPU_CONTROL_750_A2_precharge_pfc_ok2_OL SS2/updateCalib/cnt/Subsystem4 ==
  sample : Inport
  Add4 : Sum  AccumDataTypeStr=single  OutDataTypeStr=single
  Cast To Single : DataTypeConversion  OutDataTypeStr=single  SaturateOnIntegerOverflow=off  RndMeth=Floor
  Constant4 : Constant  OutDataTypeStr=single
  Data Store Read4 : DataStoreRead  DataStoreName=cnt_calib  IndexOptions=Index vector (dialog)  Indices=1  OutputSizes=1
  Delay2 : Delay  DelayLength=1
  Divide3 : Product  Inputs=*/  OutDataTypeStr=single
  Divide4 : Product  Inputs=**/  OutDataTypeStr=single
  Subtract1 : Sum  Inputs=+-  AccumDataTypeStr=single  OutDataTypeStr=single
  average : Outport
  wires:
  Constant4/1 -> Subtract1/2
  Divide4/1 -> Add4/1
  Cast To Single/1 -> Subtract1/1, Divide4/3, Divide3/2
  Divide3/1 -> Add4/2
  Subtract1/1 -> Divide4/2
  Delay2/1 -> Divide4/1
  sample/1 -> Divide3/1
  Add4/1 -> average/1, Delay2/1
  Data Store Read4/1 -> Cast To Single/1

== system npc_controller/CONTROL/STATE-MACHINE/CPU_CONTROL_750_A2_precharge_pfc_ok2_OL SS2/updateCalib/cnt/Subsystem5 ==
  sample : Inport
  Add4 : Sum  AccumDataTypeStr=single  OutDataTypeStr=single
  Cast To Single : DataTypeConversion  OutDataTypeStr=single  SaturateOnIntegerOverflow=off  RndMeth=Floor
  Constant4 : Constant  OutDataTypeStr=single
  Data Store Read4 : DataStoreRead  DataStoreName=cnt_calib  IndexOptions=Index vector (dialog)  Indices=1  OutputSizes=1
  Delay2 : Delay  DelayLength=1
  Divide3 : Product  Inputs=*/  OutDataTypeStr=single
  Divide4 : Product  Inputs=**/  OutDataTypeStr=single
  Subtract1 : Sum  Inputs=+-  AccumDataTypeStr=single  OutDataTypeStr=single
  average : Outport
  wires:
  Constant4/1 -> Subtract1/2
  Divide4/1 -> Add4/1
  Cast To Single/1 -> Subtract1/1, Divide4/3, Divide3/2
  Divide3/1 -> Add4/2
  Subtract1/1 -> Divide4/2
  Delay2/1 -> Divide4/1
  sample/1 -> Divide3/1
  Add4/1 -> average/1, Delay2/1
  Data Store Read4/1 -> Cast To Single/1

== system npc_controller/CONTROL/STATE-MACHINE/CPU_CONTROL_750_A2_precharge_pfc_ok2_OL SS2/updateCalib/cnt/Subsystem6 ==
  sample : Inport
  Add4 : Sum  AccumDataTypeStr=single  OutDataTypeStr=single
  Cast To Single : DataTypeConversion  OutDataTypeStr=single  SaturateOnIntegerOverflow=off  RndMeth=Floor
  Constant4 : Constant  OutDataTypeStr=single
  Data Store Read4 : DataStoreRead  DataStoreName=cnt_calib  IndexOptions=Index vector (dialog)  Indices=1  OutputSizes=1
  Delay2 : Delay  DelayLength=1
  Divide3 : Product  Inputs=*/  OutDataTypeStr=single
  Divide4 : Product  Inputs=**/  OutDataTypeStr=single
  Subtract1 : Sum  Inputs=+-  AccumDataTypeStr=single  OutDataTypeStr=single
  average : Outport
  wires:
  Data Store Read4/1 -> Cast To Single/1
  Add4/1 -> Delay2/1, average/1
  sample/1 -> Divide3/1
  Delay2/1 -> Divide4/1
  Subtract1/1 -> Divide4/2
  Divide3/1 -> Add4/2
  Cast To Single/1 -> Divide3/2, Divide4/3, Subtract1/1
  Divide4/1 -> Add4/1
  Constant4/1 -> Subtract1/2

== system npc_controller/CONTROL/STATE-MACHINE/CPU_CONTROL_750_A2_precharge_pfc_ok2_OL SS2/updateCalib/done/AUTO-CALIB_DONE ==
  Trigger : TriggerPort  TriggerType=function-call  VariantControl=(inherit)  PortDimensions=1
  Constant1 : Constant  OutDataTypeStr=boolean  SampleTime=-1
  Constant2 : Constant  OutDataTypeStr=uint16  SampleTime=-1
  Data Store Read : DataStoreRead  DataStoreName=adc_offset_ib_tmp  IndexOptions=Index vector (dialog)  Indices=1  OutputSizes=1
  Data Store Read1 : DataStoreRead  DataStoreName=adc_offset_ic_tmp  IndexOptions=Index vector (dialog)  Indices=1  OutputSizes=1
  Data Store Read2 : DataStoreRead  DataStoreName=adc_offset_va_tmp  IndexOptions=Index vector (dialog)  Indices=1  OutputSizes=1
  Data Store Read3 : DataStoreRead  DataStoreName=adc_offset_vb_tmp  IndexOptions=Index vector (dialog)  Indices=1  OutputSizes=1
  Data Store Read4 : DataStoreRead  DataStoreName=adc_offset_vc_tmp  IndexOptions=Index vector (dialog)  Indices=1  OutputSizes=1
  Data Store Read5 : DataStoreRead  DataStoreName=adc_offset_ia_tmp  IndexOptions=Index vector (dialog)  Indices=1  OutputSizes=1
  Data Store Write : DataStoreWrite  DataStoreName=adc_offset_ib  IndexOptions=Index vector (dialog)  Indices=1  OutputSizes=1
  Data Store Write1 : DataStoreWrite  DataStoreName=adc_offset_ic  IndexOptions=Index vector (dialog)  Indices=1  OutputSizes=1
  Data Store Write2 : DataStoreWrite  DataStoreName=cnt_calib  IndexOptions=Index vector (dialog)  Indices=1  OutputSizes=1
  Data Store Write3 : DataStoreWrite  DataStoreName=adc_offset_va  IndexOptions=Index vector (dialog)  Indices=1  OutputSizes=1
  Data Store Write4 : DataStoreWrite  DataStoreName=adc_offset_vb  IndexOptions=Index vector (dialog)  Indices=1  OutputSizes=1
  Data Store Write5 : DataStoreWrite  DataStoreName=adc_offset_vc  IndexOptions=Index vector (dialog)  Indices=1  OutputSizes=1
  Data Store Write6 : DataStoreWrite  DataStoreName=adc_offset_ia  IndexOptions=Index vector (dialog)  Indices=1  OutputSizes=1
  Scope : Scope
  Out1 : Outport
  wires:
  Data Store Read1/1 -> Data Store Write1/1
  Data Store Read3/1 -> Data Store Write4/1
  Data Store Read4/1 -> Data Store Write5/1
  Data Store Read2/1 -> Data Store Write3/1, Scope/1
  Data Store Read/1 -> Data Store Write/1
  Constant2/1 -> Data Store Write2/1
  Data Store Read5/1 -> Data Store Write6/1
  Constant1/1 -> Out1/1

== system npc_controller/CONTROL/STATE-MACHINE/CPU_CONTROL_750_A2_precharge_pfc_ok2_OL SS2/updateCalib/done/CLEAR_FAULTS ==
  Trigger : TriggerPort  TriggerType=function-call  VariantControl=(inherit)  PortDimensions=1
  Constant1 : Constant  Value=0  OutDataTypeStr=uint16  SampleTime=-1
  Constant3 : Constant  Value=0  OutDataTypeStr=boolean  SampleTime=-1
  Constant4 : Constant  Value=0  OutDataTypeStr=boolean  SampleTime=-1
  Constant5 : Constant  Value=0  OutDataTypeStr=boolean  SampleTime=-1
  Constant6 : Constant  Value=0  OutDataTypeStr=uint16  SampleTime=-1
  Constant7 : Constant  Value=0  OutDataTypeStr=uint16  SampleTime=-1
  Data Store Write1 : DataStoreWrite  DataStoreName=tz_cmpssocp  IndexOptions=Index vector (dialog)  Indices=1  OutputSizes=1
  Data Store Write10 : DataStoreWrite  DataStoreName=tz_ocp  IndexOptions=Index vector (dialog)  Indices=1  OutputSizes=1
  Data Store Write11 : DataStoreWrite  DataStoreName=tz_ovp  IndexOptions=Index vector (dialog)  Indices=1  OutputSizes=1
  Data Store Write7 : DataStoreWrite  DataStoreName=tfv_iphasea  IndexOptions=Index vector (dialog)  Indices=1  OutputSizes=1
  Data Store Write8 : DataStoreWrite  DataStoreName=tfv_iphaseb  IndexOptions=Index vector (dialog)  Indices=1  OutputSizes=1
  Data Store Write9 : DataStoreWrite  DataStoreName=tfv_iphasec  IndexOptions=Index vector (dialog)  Indices=1  OutputSizes=1
  wires:
  Constant7/1 -> Data Store Write11/1
  Constant4/1 -> Data Store Write8/1
  Constant3/1 -> Data Store Write7/1
  Constant5/1 -> Data Store Write9/1
  Constant6/1 -> Data Store Write10/1
  Constant1/1 -> Data Store Write1/1

== system npc_controller/CONTROL/STATE-MACHINE/CPU_CONTROL_750_A2_precharge_pfc_ok2_OL SS2/updateCalib/done/RESET_TZ ==
  note: //npc_controller_DWork.tz_ocp = 0b0;
      |
      | EALLOW;
      |
      | /*Disabled tripzone action*/
      | EPwm2Regs.TZCTL.bit.TZA = (uint16_T)(0b11); //do nothing
      | EPwm2Regs.TZCTL.bit.TZB = (uint16_T)(0b11);
      | EPwm7Regs.TZCTL.bit.TZA = (uint16_T)(0b11);
      | EPwm7Regs.TZCTL.bit.TZB = (uint16_T)(0b11);
      | EPwm8Regs.TZCTL.bit.TZA = (uint16_T)(0b11);
      | EPwm8Regs.TZCTL.bit.TZB = (uint16_T)(0b11);
      | EPwm9Regs.TZCTL.bit.TZA = (uint16_T)(0b11);
      | EPwm9Regs.TZCTL.bit.TZB = (uint16_T)(0b11);
      | EPwm10Regs.TZCTL.bit.TZA = (uint16_T)(0b11);
      | EPwm10Regs.TZCTL.bit.TZB = (uint16_T)(0b11);
      | EPwm11Regs.TZCTL.bit.TZA = (uint16_T)(0b11);
      | EPwm11Regs.TZCTL.bit.TZB = (uint16_T)(0b11);
      |
      | /*Clear grouped OST TZ flags*/
      | EPwm2Regs.TZCLR.bit.OST = 0b1; //clear trip
      | EPwm7Regs.TZCLR.bit.OST = 0b1;
      | EPwm8Regs.TZCLR.bit.OST = 0b1;
      | EPwm9Regs.TZCLR.bit.OST = 0b1;
      | EPwm10Regs.TZCLR.bit.OST = 0b1;
      | EPwm11Regs.TZCLR.bit.OST = 0b1;
      |
      | /*Clear individual OST TZ flags*/
      | EPwm2Regs.TZOSTCLR.bit.OST1 = 0b1; //clear trip
      | EPwm2Regs.TZOSTCLR.bit.OST2 = 0b1;
      | EPwm7Regs.TZOSTCLR.bit.OST1 = 0b1;
      | EPwm7Regs.TZOSTCLR.bit.OST2 = 0b1;
      | EPwm8Regs.TZOSTCLR.bit.OST1 = 0b1;
      | EPwm8Regs.TZOSTCLR.bit.OST2 = 0b1;
      | EPwm9Regs.TZOSTCLR.bit.OST1 = 0b1;
      | EPwm9Regs.TZOSTCLR.bit.OST2 = 0b1;
      | EPwm10Regs.TZOSTCLR.bit.OST1 = 0b1;
      | EPwm10Regs.TZOSTCLR.bit.OST2 = 0b1;
      | EPwm11Regs.TZOSTCLR.bit.OST1 = 0b1;
      | EPwm11Regs.TZOSTCLR.bit.OST2 = 0b1;
      |
      | /*Enable tripzone action*/
      | EPwm2Regs.TZCTL.bit.TZA = (uint16_T)(0b10); //force to LOW
      | EPwm2Regs.TZCTL.bit.TZB = (uint16_T)(0b10);
      | EPwm7Regs.TZCTL.bit.TZA = (uint16_T)(0b10);
      | EPwm7Regs.TZCTL.bit.TZB = (uint16_T)(0b10);
      | EPwm8Regs.TZCTL.bit.TZA = (uint16_T)(0b10);
      | EPwm8Regs.TZCTL.bit.TZB = (uint16_T)(0b10);
      | EPwm9Regs.TZCTL.bit.TZA = (uint16_T)(0b10);
      | EPwm9Regs.TZCTL.bit.TZB = (uint16_T)(0b10);
      | EPwm10Regs.TZCTL.bit.TZA = (uint16_T)(0b10);
      | EPwm10Regs.TZCTL.bit.TZB = (uint16_T)(0b10);
      | EPwm11Regs.TZCTL.bit.TZA = (uint16_T)(0b10);
      | EPwm11Regs.TZCTL.bit.TZB = (uint16_T)(0b10);
      |
      | EDIS;
  note: Note:
      | TZCCTL
      | 0b00 - High impedance
      | 0b01 - Force to HIGH
      | 0b10 - Force to LOW
      | 0b11 - Do nothing
      |
      | AQCSFRC
      | 0b00 - disables forced PWM
      | 0b01 - forces PWM to LOW
      | 0b10 - forces PWM to  HIGH
  note: //npc_controller_DWork.tz_ocp = 0b0;
      |
      | EALLOW;
      |
      | /*Disabled tripzone action*/
      | EPwm2Regs.TZCTL.bit.TZA = (uint16_T)(0b11); //do nothing
      | EPwm2Regs.TZCTL.bit.TZB = (uint16_T)(0b11);
      | EPwm7Regs.TZCTL.bit.TZA = (uint16_T)(0b11);
      | EPwm7Regs.TZCTL.bit.TZB = (uint16_T)(0b11);
      | EPwm8Regs.TZCTL.bit.TZA = (uint16_T)(0b11);
      | EPwm8Regs.TZCTL.bit.TZB = (uint16_T)(0b11);
      | EPwm9Regs.TZCTL.bit.TZA = (uint16_T)(0b11);
      | EPwm9Regs.TZCTL.bit.TZB = (uint16_T)(0b11);
      | EPwm10Regs.TZCTL.bit.TZA = (uint16_T)(0b11);
      | EPwm10Regs.TZCTL.bit.TZB = (uint16_T)(0b11);
      | EPwm11Regs.TZCTL.bit.TZA = (uint16_T)(0b11);
      | EPwm11Regs.TZCTL.bit.TZB = (uint16_T)(0b11);
      |
      | /*Disabled Digital Compare Out A and Out B Event1*/
      | //EPwm2Regs.TZCTL.bit.DCAEVT1 = 0b11; //do nothing
      | //EPwm2Regs.TZCTL.bit.DCBEVT1 = 0b11;
      | //EPwm7Regs.TZCTL.bit.DCAEVT1 = 0b11;
      | //EPwm7Regs.TZCTL.bit.DCBEVT1 = 0b11;
      |
      | //EPwm8Regs.TZCTL.bit.DCAEVT1 = 0b11;
      | //EPwm8Regs.TZCTL.bit.DCBEVT1 = 0b11;
      | //EPwm9Regs.TZCTL.bit.DCAEVT1 = 0b11;
      | //EPwm9Regs.TZCTL.bit.DCBEVT1 = 0b11;
      |
      | //EPwm10Regs.TZCTL.bit.DCAEVT1 = 0b11;
      | //EPwm10Regs.TZCTL.bit.DCBEVT1 = 0b11;
      | //EPwm11Regs.TZCTL.bit.DCAEVT1 = 0b11;
      | //EPwm11Regs.TZCTL.bit.DCBEVT1 = 0b11;
      |
      | /*Disabled Digital Compare Out A and Out B Event1 */
      | EPwm2Regs.TZSEL.bit.DCAEVT1 = 0b0; //disable DCAEVT1 for the ePWM module
      | EPwm2Regs.TZSEL.bit.DCBEVT1 = 0b0;
      | EPwm7Regs.TZSEL.bit.DCAEVT1 = 0b0;
      | EPwm7Regs.TZSEL.bit.DCBEVT1 = 0b0;
      |
      | EPwm8Regs.TZSEL.bit.DCAEVT1 = 0b0;
      | EPwm8Regs.TZSEL.bit.DCBEVT1 = 0b0;
      | EPwm9Regs.TZSEL.bit.DCAEVT1 = 0b0;
      | EPwm9Regs.TZSEL.bit.DCBEVT1 = 0b0;
      |
      | EPwm10Regs.TZSEL.bit.DCAEVT1 = 0b0;
      | EPwm10Regs.TZSEL.bit.DCBEVT1 = 0b0;
      | EPwm11Regs.TZSEL.bit.DCAEVT1 = 0b0;
      | EPwm11Regs.TZSEL.bit.DCBEVT1 = 0b0;
      |
      | /*Clear grouped OST TZ flags*/
      | EPwm2Regs.TZCLR.bit.OST = 0b1; //clear trip
      | EPwm7Regs.TZCLR.bit.OST = 0b1;
      | EPwm8Regs.TZCLR.bit.OST = 0b1;
      | EPwm9Regs.TZCLR.bit.OST = 0b1;
      | EPwm10Regs.TZCLR.bit.OST = 0b1;
      | EPwm11Regs.TZCLR.bit.OST = 0b1;
      |
      | /*Clear Digital Compare Out A and B Event1 flags */
      | EPwm2Regs.TZCLR.bit.DCAEVT1 = 0b1; //clear trip
      | EPwm2Regs.TZCLR.bit.DCBEVT1 = 0b1;
      | EPwm7Regs.TZCLR.bit.DCAEVT1 = 0b1;
      | EPwm7Regs.TZCLR.bit.DCBEVT1 = 0b1;
      |
      | EPwm8Regs.TZCLR.bit.DCAEVT1 = 0b1;
      | EPwm8Regs.TZCLR.bit.DCBEVT1 = 0b1;
      | EPwm9Regs.TZCLR.bit.DCAEVT1 = 0b1;
      | EPwm9Regs.TZCLR.bit.DCBEVT1 = 0b1;
      |
      | EPwm10Regs.TZCLR.bit.DCAEVT1 = 0b1;
      | EPwm10Regs.TZCLR.bit.DCBEVT1 = 0b1;
      | EPwm11Regs.TZCLR.bit.DCAEVT1 = 0b1;
      | EPwm11Regs.TZCLR.bit.DCBEVT1 = 0b1;
      |
      | /*Enabled Digital Compare Out A and Out B Event1 */
      | EPwm2Regs.TZSEL.bit.DCAEVT1 = 0b1; //enabled DCAEVT1 for the ePWM module
      | EPwm2Regs.TZSEL.bit.DCBEVT1 = 0b1;
      | EPwm7Regs.TZSEL.bit.DCAEVT1 = 0b1;
      | EPwm7Regs.TZSEL.bit.DCBEVT1 = 0b1;
      |
      | EPwm8Regs.TZSEL.bit.DCAEVT1 = 0b1;
      | EPwm8Regs.TZSEL.bit.DCBEVT1 = 0b1;
      | EPwm9Regs.TZSEL.bit.DCAEVT1 = 0b1;
      | EPwm9Regs.TZSEL.bit.DCBEVT1 = 0b1;
      |
      | EPwm10Regs.TZSEL.bit.DCAEVT1 = 0b1;
      | EPwm10Regs.TZSEL.bit.DCBEVT1 = 0b1;
      | EPwm11Regs.TZSEL.bit.DCAEVT1 = 0b1;
      | EPwm11Regs.TZSEL.bit.DCBEVT1 = 0b1;
      |
      | /*Clear individual OST TZ flags*/
      | EPwm2Regs.TZOSTCLR.bit.OST1 = 0b1; //clear trip
      | EPwm2Regs.TZOSTCLR.bit.OST2 = 0b1;
      | EPwm7Regs.TZOSTCLR.bit.OST1 = 0b1;
      | EPwm7Regs.TZOSTCLR.bit.OST2 = 0b1;
      | EPwm8Regs.TZOSTCLR.bit.OST1 = 0b1;
      | EPwm8Regs.TZOSTCLR.bit.OST2 = 0b1;
      | EPwm9Regs.TZOSTCLR.bit.OST1 = 0b1;
      | EPwm9Regs.TZOSTCLR.bit.OST2 = 0b1;
      | EPwm10Regs.TZOSTCLR.bit.OST1 = 0b1;
      | EPwm10Regs.TZOSTCLR.bit.OST2 = 0b1;
      | EPwm11Regs.TZOSTCLR.bit.OST1 = 0b1;
      | EPwm11Regs.TZOSTCLR.bit.OST2 = 0b1;
      |
      | /*Enable tripzone action*/
      | EPwm2Regs.TZCTL.bit.TZA = (uint16_T)(0b10); //force to LOW
      | EPwm2Regs.TZCTL.bit.TZB = (uint16_T)(0b10);
      | EPwm7Regs.TZCTL.bit.TZA = (uint16_T)(0b10);
      | EPwm7Regs.TZCTL.bit.TZB = (uint16_T)(0b10);
      | EPwm8Regs.TZCTL.bit.TZA = (uint16_T)(0b10);
      | EPwm8Regs.TZCTL.bit.TZB = (uint16_T)(0b10);
      | EPwm9Regs.TZCTL.bit.TZA = (uint16_T)(0b10);
      | EPwm9Regs.TZCTL.bit.TZB = (uint16_T)(0b10);
      | EPwm10Regs.TZCTL.bit.TZA = (uint16_T)(0b10);
      | EPwm10Regs.TZCTL.bit.TZB = (uint16_T)(0b10);
      | EPwm11Regs.TZCTL.bit.TZA = (uint16_T)(0b10);
      | EPwm11Regs.TZCTL.bit.TZB = (uint16_T)(0b10);
      |
      | /*Enabled Digital Compare Out A and Out B Event1*/
      | //EPwm2Regs.TZCTL.bit.DCAEVT1 = 0b10; //force to LOW
      | //EPwm2Regs.TZCTL.bit.DCBEVT1 = 0b10;
      | //EPwm7Regs.TZCTL.bit.DCAEVT1 = 0b10;
      | //EPwm7Regs.TZCTL.bit.DCBEVT1 = 0b10;
      |
      | //EPwm8Regs.TZCTL.bit.DCAEVT1 = 0b10;
      | //EPwm8Regs.TZCTL.bit.DCBEVT1 = 0b10;
      | //EPwm9Regs.TZCTL.bit.DCAEVT1 = 0b10;
      | //EPwm9Regs.TZCTL.bit.DCBEVT1 = 0b10;
      |
      | //EPwm10Regs.TZCTL.bit.DCAEVT1 = 0b10;
      | //EPwm10Regs.TZCTL.bit.DCBEVT1 = 0b10;
      | //EPwm11Regs.TZCTL.bit.DCAEVT1 = 0b10;
      | //EPwm11Regs.TZCTL.bit.DCBEVT1 = 0b10;
      |
      | EDIS;
  Trigger : TriggerPort  TriggerType=function-call  VariantControl=(inherit)  PortDimensions=1
  System Outputs1 : Subsystem  mask(System Outputs){ShowInLibBrowser=0}
      mask prompts: ShowInLibBrowser "Simulink:masks:CustCodeMaskParam1_MP"
      settings: CopyFcn=cccopyfcn(gcb)  OpenFcn=ccopenfcn('System Outputs Function')
      mask Help: eval('feval(''rtwprivate'',''rtwhelpview'',''rtw_sys_outputs_block'')');
      mask Display: disp('System\nOutputs');
  System Outputs2 : Subsystem  Commented=on  mask(System Outputs){ShowInLibBrowser=0}
      mask prompts: ShowInLibBrowser "Simulink:masks:CustCodeMaskParam1_MP"
      settings: CopyFcn=cccopyfcn(gcb)  OpenFcn=ccopenfcn('System Outputs Function')
      mask Help: eval('feval(''rtwprivate'',''rtwhelpview'',''rtw_sys_outputs_block'')');
      mask Display: disp('System\nOutputs');

== system npc_controller/CONTROL/STATE-MACHINE/CPU_CONTROL_750_A2_precharge_pfc_ok2_OL SS2/updatePll3p/PLL/SRF_PLL ==
  Vabc : Inport
  Demux1 : Demux  Outputs=3
  Gain : Gain  Commented=on  Gain=1/(2*pi)
  Integrator : Subsystem
  Memory : Memory  InheritSampleTime=on  LinearizeAsDelay=on
  PI : Subsystem
  Subsystem1 : Subsystem  Commented=on
  Sum1 : Sum  Inputs=|++  AccumDataTypeStr=single  OutDataTypeStr=single
  abc to dq : Subsystem
  f0 : Constant  Value=2*pi*50  OutDataTypeStr=fixdt('single', 'DataTypeOverride', 'Off')
  SinVal : Outport  VectorParamsAs1DForOutWhenUnconnected=off
  CosVal : Outport  Port=2  VectorParamsAs1DForOutWhenUnconnected=off
  theta : Outport  Port=3  OutDataTypeStr=single  VectorParamsAs1DForOutWhenUnconnected=off
  wires:
  Demux1/3 -> abc to dq/3(c)
  Demux1/2 -> abc to dq/2(b)
  Demux1/1 -> abc to dq/1(a)
  Sum1/1 -> Integrator/1(PI Out), Gain/1
  PI/1(PI Out) -> Sum1/1
  Gain/1 -> Subsystem1/1(x[n])  "Freq_Unf"
  f0/1 -> Sum1/2
  abc to dq/1(q) -> PI/1(Vq)
  Integrator/1(wt) -> theta/1, Memory/1
  Memory/1 -> abc to dq/4(wt)
  Vabc/1 -> Demux1/1

== system npc_controller/CONTROL/STATE-MACHINE/CPU_CONTROL_750_A2_precharge_pfc_ok2_OL SS2/updatePll3p/PLL/Subsystem ==
  In1 : Inport
  Cast To Single : DataTypeConversion  OutDataTypeStr=single  SaturateOnIntegerOverflow=off  RndMeth=Floor
  Constant2 : Constant  Value=0
  GreaterThan1 : RelationalOperator  Operator=>  OutDataTypeStr=boolean  RndMeth=Simplest  InputSameDT=off
  Initialize at Zero Crossing : Subsystem  TreatAsAtomicUnit=on
  Out1 : Outport
  wires:
  Cast To Single/1 -> Out1/1
  In1/1 -> GreaterThan1/1
  Initialize at Zero Crossing/1(Out1) -> Cast To Single/1
  Constant2/1 -> GreaterThan1/2
  GreaterThan1/1 -> Initialize at Zero Crossing/1(In1), Initialize at Zero Crossing/Trigger

== system npc_controller/CONTROL/STATE-MACHINE/CPU_CONTROL_750_A2_precharge_pfc_ok2_OL SS2/updateSequencePhA/pol_final1/pol_vxn ==
  vxn : Inport
  Action Port : ActionPort
  Out1 : Outport
  wires:
  vxn/1 -> Out1/1

== system npc_controller/CONTROL/STATE-MACHINE/CPU_CONTROL_750_A2_precharge_pfc_ok2_OL SS2/updateSequencePhA/pol_final1/prot ==
  note: Note:
      | AQCSFRC
      | 0b00 - disables forced PWM
      | 0b01 - forces PWM to LOW
      | 0b10 - forces PWM to  HIGH
  note: /*Force PWM to LOW*/
      | EPwm6Regs.AQCSFRC.bit.CSFA = (uint16_T)(0b01);
      | EPwm6Regs.AQCSFRC.bit.CSFB = (uint16_T)(0b01);
      | EPwm7Regs.AQCSFRC.bit.CSFA = (uint16_T)(0b01);
      | EPwm7Regs.AQCSFRC.bit.CSFB = (uint16_T)(0b01);
      | EPwm8Regs.AQCSFRC.bit.CSFA = (uint16_T)(0b01);
      | EPwm8Regs.AQCSFRC.bit.CSFB = (uint16_T)(0b01);
      | EPwm9Regs.AQCSFRC.bit.CSFA = (uint16_T)(0b01);
      | EPwm9Regs.AQCSFRC.bit.CSFB = (uint16_T)(0b01);
      | EPwm10Regs.AQCSFRC.bit.CSFA = (uint16_T)(0b01);
      | EPwm10Regs.AQCSFRC.bit.CSFB = (uint16_T)(0b01);
      | EPwm11Regs.AQCSFRC.bit.CSFA = (uint16_T)(0b01);
      | EPwm11Regs.AQCSFRC.bit.CSFB = (uint16_T)(0b01);
  note: Note:
      |
      | Function PWM # GPIO # LAUNCHPAD PIN #
      |
      | Synci EPWM1A GPIO0 J4.40
      | EPWM1B GPIO1 J4.39
      |
      | TZ GPIO62 XX
      |
      | a_s1 EPWM6B GPIO11 J8.75
      | a_s2 EPWM7B GPIO13 XX
      | a_s3 EPWM6A GPIO10 J8.76
      | a_s4 EPWM7A GPIO12 XX
      |
      | b_s1 EPWM8B GPIO15 J8.73
      | b_s2 EPWM9B GPIO17 XX
      | b_s3 EPWM8A GPIO14 J8.74
      | b_s4 EPWM9A GPIO16 J4.33
      |
      | c_s1 EPWM10B GPIO19 J1.3
      | c_s2 EPWM11B GPIO21 XX
      | c_s3 EPWM10A GPIO18 J1.4
      | c_s4 EPWM11A GPIO20 XX
  Action Port : ActionPort
  Constant : Constant  Value=0  OutDataTypeStr=uint8  SampleTime=-1
  System Outputs : Subsystem  mask(System Outputs){ShowInLibBrowser=0}
      mask prompts: ShowInLibBrowser "Simulink:masks:CustCodeMaskParam1_MP"
      settings: CopyFcn=cccopyfcn(gcb)  OpenFcn=ccopenfcn('System Outputs Function')
      mask Help: eval('feval(''rtwprivate'',''rtwhelpview'',''rtw_sys_outputs_block'')');
      mask Display: disp('System\nOutputs');
  Out1 : Outport
  wires:
  Constant/1 -> Out1/1

== system npc_controller/CONTROL/STATE-MACHINE/CPU_CONTROL_750_A2_precharge_pfc_ok2_OL SS2/updateSequencePhA/pol_ix1/neg ==
  Action Port : ActionPort
  Constant : Constant  Value=2  OutDataTypeStr=uint8  SampleTime=-1
  Out1 : Outport
  wires:
  Constant/1 -> Out1/1

== system npc_controller/CONTROL/STATE-MACHINE/CPU_CONTROL_750_A2_precharge_pfc_ok2_OL SS2/updateSequencePhA/pol_ix1/pos ==
  Action Port : ActionPort
  Constant : Constant  OutDataTypeStr=uint8  SampleTime=-1
  Out1 : Outport
  wires:
  Constant/1 -> Out1/1

== system npc_controller/CONTROL/STATE-MACHINE/CPU_CONTROL_750_A2_precharge_pfc_ok2_OL SS2/updateSequencePhA/pol_ix1/zero ==
  Action Port : ActionPort
  Constant : Constant  Value=0  OutDataTypeStr=uint8  SampleTime=-1
  Out1 : Outport
  wires:
  Constant/1 -> Out1/1

== system npc_controller/CONTROL/STATE-MACHINE/CPU_CONTROL_750_A2_precharge_pfc_ok2_OL SS2/updateSequencePhA/pol_vxn1/neg ==
  note: 48digital = 2A
  ixn : Inport
  Action Port : ActionPort  ActionPortLabel=else
  If : If  IfExpression="(u1 > -48)  & (u1 < 48)"
  Merge : Merge
  SR OFF : Subsystem  TreatAsAtomicUnit=on
  SR ON : Subsystem  TreatAsAtomicUnit=on
  Out1 : Outport
  wires:
  ixn/1 -> If/1
  If/2 -> SR ON/Action
  If/1 -> SR OFF/Action
  Merge/1 -> Out1/1
  SR OFF/1(Out1) -> Merge/1
  SR ON/1(Out1) -> Merge/2

== system npc_controller/CONTROL/STATE-MACHINE/CPU_CONTROL_750_A2_precharge_pfc_ok2_OL SS2/updateSequencePhA/pol_vxn1/pos ==
  note: 48digital = 2A
  ixn : Inport
  Action Port : ActionPort  ActionPortLabel=elseif(u1 >= 16)
  If : If  IfExpression="(u1 > -48)  & (u1 < 48)"
  Merge : Merge
  SR Force to Low : Subsystem  TreatAsAtomicUnit=on
  SR ON : Subsystem  TreatAsAtomicUnit=on
  Out1 : Outport
  wires:
  ixn/1 -> If/1
  If/1 -> SR Force to Low/Action
  If/2 -> SR ON/Action
  SR Force to Low/1(Out1) -> Merge/1
  SR ON/1(Out1) -> Merge/2
  Merge/1 -> Out1/1

== system npc_controller/CONTROL/STATE-MACHINE/CPU_CONTROL_750_A2_precharge_pfc_ok2_OL SS2/updateSequencePhA/pol_vxn1/zero ==
  note: Note:
      |
      | Function PWM # GPIO # LAUNCHPAD PIN #
      |
      | Synci EPWM1A GPIO0 J4.40
      | EPWM1B GPIO1 J4.39
      |
      | ORPS EPMW2A GPIO2 J4.38
      | EPWM2B GPIO3 J4.37
      |
      | RELAY EPWM3A GPIO4 J4.36
      |
      | TZ GPIO62 XX
      |
      | a_s1 EPWM6A GPIO10 J8.76
      | a_s2 EPWM7B GPIO13 XX
      | a_s3 EPWM6B GPIO11 J8.75
      | a_s4 EPWM7A GPIO12 XX
      |
      | b_s1 EPWM8B GPIO15 J8.73
      | b_s2 EPWM9B GPIO17 XX
      | b_s3 EPWM8A GPIO14 J8.74
      | b_s4 EPWM9A GPIO16 J4.33
      |
      | c_s1 EPWM10B GPIO19 J1.3
      | c_s2 EPWM11B GPIO21 XX
      | c_s3 EPWM10A GPIO18 J1.4
      | c_s4 EPWM11A GPIO20 XX
  note: Note:
      | AQCSFRC
      | 0b00 - disables forced PWM
      | 0b01 - forces PWM to LOW
      | 0b10 - forces PWM to  HIGH
  note: /*Force PWM to LOW*/
      | EPwm2Regs.AQCSFRC.bit.CSFA = (uint16_T)(0b01);
      | EPwm7Regs.AQCSFRC.bit.CSFB = (uint16_T)(0b01);
      | EPwm2Regs.AQCSFRC.bit.CSFB = (uint16_T)(0b01);
      | EPwm7Regs.AQCSFRC.bit.CSFA = (uint16_T)(0b01);
  Action Port : ActionPort  ActionPortLabel="if((u1 > -16)  & (u1 < 16))"
  Constant : Constant  Value=0  OutDataTypeStr=uint8  SampleTime=-1
  System Outputs1 : Subsystem  mask(System Outputs){ShowInLibBrowser=0}
      mask prompts: ShowInLibBrowser "Simulink:masks:CustCodeMaskParam1_MP"
      settings: CopyFcn=cccopyfcn(gcb)  OpenFcn=ccopenfcn('System Outputs Function')
      mask Help: eval('feval(''rtwprivate'',''rtwhelpview'',''rtw_sys_outputs_block'')');
      mask Display: disp('System\nOutputs');
  Out1 : Outport
  wires:
  Constant/1 -> Out1/1
